simulink model "Modelo_Cinematico_Spline"  (R2020b)
settings: Solver=VariableStepAuto  StartTime=0.0  StopTime=290  RelTol=1e-3
undefined symbols (not defined in the file or in its folder): magnitude
libraries: simulink x2
settings Model: Creator=danie  LastModifiedBy=danie

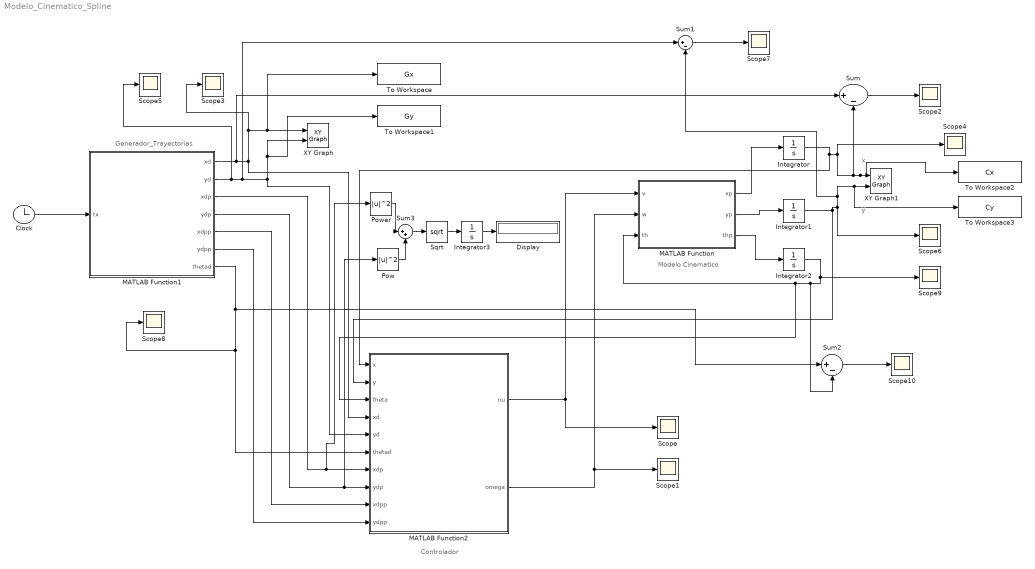
== system Modelo_Cinematico_Spline ==
  note: y
  note: x
  note: Controlador
  note: Generador_Trayectorias
  note: Modelo Cinematico
  Clock : Clock
  Display : Display
  Integrator : Integrator  InitialCondition=50.0557
  Integrator1 : Integrator  InitialCondition=50.0866
  Integrator2 : Integrator
  Integrator3 : Integrator
  MATLAB Function : MATLAB Function  TreatAsAtomicUnit=on
  MATLAB Function1 : MATLAB Function  TreatAsAtomicUnit=on
  MATLAB Function2 : MATLAB Function  TreatAsAtomicUnit=on
  Pow : Math  Operator=magnitude^2  SignedPower=on  RndMeth=Zero  SaturateOnIntegerOverflow=on
  Power : Math  Operator=magnitude^2  SaturateOnIntegerOverflow=on
  Scope{,1..10} (11 alike) : Scope
  Sqrt : Sqrt  SaturateOnIntegerOverflow=on
  Sum : Sum  Inputs=|+-
  Sum1 : Sum  Inputs=|+-
  Sum2 : Sum  Inputs=|+-
  Sum3 : Sum  Inputs=|++
  To Workspace : ToWorkspace  VariableName=Gx  SampleTime=-1
  To Workspace1 : ToWorkspace  VariableName=Gy  SampleTime=-1
  To Workspace2 : ToWorkspace  VariableName=Cx  SampleTime=-1
  To Workspace3 : ToWorkspace  VariableName=Cy  SampleTime=-1
  XY Graph : simulink/Sinks/XY Graph  xmin=0  xmax=100  ymin=0  ymax=100  st=-1
  XY Graph1 : simulink/Sinks/XY Graph  xmin=0  xmax=100  ymin=0  ymax=100  st=-1
  wires:
  MATLAB Function/3(thp) -> Integrator2/1
  Integrator2/1 -> Sum2/2, MATLAB Function2/3(theta), MATLAB Function/3(th), Scope9/1
  MATLAB Function/1(xp) -> Integrator/1
  MATLAB Function/2(yp) -> Integrator1/1
  MATLAB Function2/1(nu) -> MATLAB Function/1(v), Scope/1
  MATLAB Function2/2(omega) -> MATLAB Function/2(w), Scope1/1
  Integrator/1 -> MATLAB Function2/1(x), To Workspace2/1, XY Graph1/1, Sum/2, Scope4/1
  Integrator1/1 -> Scope6/1, Sum1/2, To Workspace3/1, XY Graph1/2, MATLAB Function2/2(y)
  MATLAB Function1/1(xd) -> Sum/1, MATLAB Function2/4(xd), Scope3/1, To Workspace/1, XY Graph/1
  MATLAB Function1/2(yd) -> Scope5/1, Sum1/1, To Workspace1/1, XY Graph/2, MATLAB Function2/5(yd)
  MATLAB Function1/3(xdp) -> Power/1, MATLAB Function2/7(xdp)
  MATLAB Function1/4(ydp) -> Pow/1, MATLAB Function2/8(ydp)
  MATLAB Function1/5(xdpp) -> MATLAB Function2/9(xdpp)
  MATLAB Function1/6(ydpp) -> MATLAB Function2/10(ydpp)
  MATLAB Function1/7(thetad) -> Sum2/1, Scope8/1, MATLAB Function2/6(thetad)
  Clock/1 -> MATLAB Function1/1(tx)
  Sum/1 -> Scope2/1
  Sum1/1 -> Scope7/1
  Sum2/1 -> Scope10/1
  Sum3/1 -> Sqrt/1
  Sqrt/1 -> Integrator3/1
  Integrator3/1 -> Display/1
  Power/1 -> Sum3/1
  Pow/1 -> Sum3/2

== matlab function Modelo_Cinematico_Spline/MATLAB Function1 ==
  data: xd output; yd output; tx input; xdp output; ydp output; xdpp output; ydpp output; thetad output
function [xd, yd, xdp, ydp, xdpp, ydpp, thetad] = fcn(tx)

tmax=300;

xd=(5383481803376765*sin((28386324213466055*((2*pi*tx)/tmax))/9007199254740992))/1125899906842624 - (2564781378595497*cos((28386324213466055*((2*pi*tx)/tmax))/9007199254740992))/18014398509481984 + (4975098477569247*cos((5677264842693211*((2*pi*tx)/tmax))/9007199254740992))/140737488355328 - (5532462661087593*cos((5677264842693211*((2*pi*tx)/tmax))/4503599627370496))/2251799813685248 - (4982669448405143*cos((5677264842693211*((2*pi*tx)/tmax))/2251799813685248))/281474976710656 + (6597269238774799*sin((5677264842693211*((2*pi*tx)/tmax))/9007199254740992))/562949953421312 + (7427178311913285*sin((5677264842693211*((2*pi*tx)/tmax))/4503599627370496))/2251799813685248 + (1488767062451517*sin((5677264842693211*((2*pi*tx)/tmax))/2251799813685248))/281474976710656 - (2110113036993915*cos((17031794528079633*((2*pi*tx)/tmax))/9007199254740992))/140737488355328 - (6032332211127941*sin((17031794528079633*((2*pi*tx)/tmax))/9007199254740992))/281474976710656 + 50;

yd=(2688302397518191*cos((10047744804514215*((2*pi*tx)/tmax))/4503599627370496))/281474976710656 - (773246555679083*sin((10047744804514215*((2*pi*tx)/tmax))/4503599627370496))/35184372088832 + (2417259064448069*cos((16746241340857025*((2*pi*tx)/tmax))/4503599627370496))/281474976710656 + (1557044084674199*sin((16746241340857025*((2*pi*tx)/tmax))/4503599627370496))/1125899906842624 - (826401745574083*cos((3349248268171405*((2*pi*tx)/tmax))/4503599627370496))/140737488355328 - (2589504683792575*cos((3349248268171405*((2*pi*tx)/tmax))/2251799813685248))/140737488355328 + (7002517856441785*cos((3349248268171405*((2*pi*tx)/tmax))/1125899906842624))/1125899906842624 - (5133657206379779*sin((3349248268171405*((2*pi*tx)/tmax))/4503599627370496))/1125899906842624 + (1324039837451005*sin((3349248268171405*((2*pi*tx)/tmax))/2251799813685248))/281474976710656 + (6400066323978353*sin((3349248268171405*((2*pi*tx)/tmax))/1125899906842624))/562949953421312 + 50;

xdp=(37454444707077569124597075189589*pi*cos((5677264842693211*pi*tx)/(4503599627370496*tmax)))/(2535301200456458802993406410752*tmax) + (42166058310638804388005690208135*pi*cos((5677264842693211*pi*tx)/(2251799813685248*tmax)))/(5070602400912917605986812821504*tmax) + (8452124902615645497794392551087*pi*cos((5677264842693211*pi*tx)/(1125899906842624*tmax)))/(316912650057057350374175801344*tmax) - (6421340171565460806896461762357*pi*cos((1064487158004977*pi*tx)/(281474976710656*tmax)))/(79228162514264337593543950336*tmax) - (28244951675640404604248229282117*pi*sin((5677264842693211*pi*tx)/(4503599627370496*tmax)))/(633825300114114700748351602688*tmax) + (31409255759305517195060497431123*pi*sin((5677264842693211*pi*tx)/(2251799813685248*tmax)))/(5070602400912917605986812821504*tmax) + (28287934082192092596880783584173*pi*sin((5677264842693211*pi*tx)/(1125899906842624*tmax)))/(316912650057057350374175801344*tmax) + (2246188229818903474228688714955*pi*sin((1064487158004977*pi*tx)/(281474976710656*tmax)))/(39614081257132168796771975168*tmax) + (19102157483493471684558188323605*pi*cos((3548290526683257*pi*tx)/(562949953421312*tmax)))/(633825300114114700748351602688*tmax) + (9100589468684026021756445493729*pi*sin((3548290526683257*pi*tx)/(562949953421312*tmax)))/(10141204801825835211973625643008*tmax);

ydp=(407416187817311810543913761309*pi*cos((261660020950891*pi*tx)/(35184372088832*tmax)))/(39614081257132168796771975168*tmax) - (632500057447212912553468779479*pi*sin((261660020950891*pi*tx)/(35184372088832*tmax)))/(9903520314283042199192993792*tmax) - (17193892507853127879432298019495*pi*cos((3349248268171405*pi*tx)/(2251799813685248*tmax)))/(2535301200456458802993406410752*tmax) + (4434538132572727079447629512025*pi*cos((3349248268171405*pi*tx)/(1125899906842624*tmax)))/(316912650057057350374175801344*tmax) + (21435411051766629023004113595965*pi*cos((3349248268171405*pi*tx)/(562949953421312*tmax)))/(316912650057057350374175801344*tmax) + (2767824615177823544638369696615*pi*sin((3349248268171405*pi*tx)/(2251799813685248*tmax)))/(316912650057057350374175801344*tmax) + (8672894077614023540335566317875*pi*sin((3349248268171405*pi*tx)/(1125899906842624*tmax)))/(158456325028528675187087900672*tmax) - (23453170803526987627261784157925*pi*sin((3349248268171405*pi*tx)/(562949953421312*tmax)))/(633825300114114700748351602688*tmax) - (971173007804127331951225917991*pi*cos((1255968100564277*pi*tx)/(281474976710656*tmax)))/(9903520314283042199192993792*tmax) - (3376422055953314277671472262907*pi*sin((1255968100564277*pi*tx)/(281474976710656*tmax)))/(79228162514264337593543950336*tmax);

xdpp=(32291535398964944679140506992381246790162795353*pi^2*cos((3548290526683257*pi*tx)/(562949953421312*tmax)))/(5708990770823839524233143877797980545530986496*tmax^2) - (67780004437891569776866379107147617745651381485*pi^2*sin((3548290526683257*pi*tx)/(562949953421312*tmax)))/(356811923176489970264571492362373784095686656*tmax^2) - (160354071131681968090375756460233262699399607687*pi^2*cos((5677264842693211*pi*tx)/(4503599627370496*tmax)))/(2854495385411919762116571938898990272765493248*tmax^2) + (178318663457464468702307355009051006962292205953*pi^2*cos((5677264842693211*pi*tx)/(2251799813685248*tmax)))/(11417981541647679048466287755595961091061972992*tmax^2) + (160598093637252212663730214209012445414834149503*pi^2*cos((5677264842693211*pi*tx)/(1125899906842624*tmax)))/(356811923176489970264571492362373784095686656*tmax^2) + (2391038525104154692777831774840356231624331035*pi^2*cos((1064487158004977*pi*tx)/(281474976710656*tmax)))/(11150372599265311570767859136324180752990208*tmax^2) - (212638802138088304827737641160315177219188180279*pi^2*sin((5677264842693211*pi*tx)/(4503599627370496*tmax)))/(11417981541647679048466287755595961091061972992*tmax^2) - (239387880401941574160516267743202310404541471485*pi^2*sin((5677264842693211*pi*tx)/(2251799813685248*tmax)))/(11417981541647679048466287755595961091061972992*tmax^2) - (47984951555671583979630787606204462637985570357*pi^2*sin((5677264842693211*pi*tx)/(1125899906842624*tmax)))/(356811923176489970264571492362373784095686656*tmax^2) + (6835434149812908795327482680102998001597250789*pi^2*sin((1064487158004977*pi*tx)/(281474976710656*tmax)))/(22300745198530623141535718272648361505980416*tmax^2);

ydpp=(1219762317931045568593540067381353994426207507*pi^2*sin((1255968100564277*pi*tx)/(281474976710656*tmax)))/(2787593149816327892691964784081045188247552*tmax^2) - (4240678396319015130497079762907630620796373239*pi^2*cos((1255968100564277*pi*tx)/(281474976710656*tmax)))/(22300745198530623141535718272648361505980416*tmax^2) - (165499978283077491769036625538731210767565789*pi^2*cos((261660020950891*pi*tx)/(35184372088832*tmax)))/(348449143727040986586495598010130648530944*tmax^2) - (106604528240009950942948130502300866584876319*pi^2*sin((261660020950891*pi*tx)/(35184372088832*tmax)))/(1393796574908163946345982392040522594123776*tmax^2) + (9270131798986510997054235237400213970668294075*pi^2*cos((3349248268171405*pi*tx)/(2251799813685248*tmax)))/(713623846352979940529142984724747568191373312*tmax^2) + (29047675469482803324353555333873198935215364375*pi^2*cos((3349248268171405*pi*tx)/(1125899906842624*tmax)))/(178405961588244985132285746181186892047843328*tmax^2) - (78550491696840922343442503487770950837489134625*pi^2*cos((3349248268171405*pi*tx)/(562949953421312*tmax)))/(356811923176489970264571492362373784095686656*tmax^2) + (57586614705052384093879702349227552026691540475*pi^2*sin((3349248268171405*pi*tx)/(2251799813685248*tmax)))/(5708990770823839524233143877797980545530986496*tmax^2) - (14852369160659262563490299824908137359208645125*pi^2*sin((3349248268171405*pi*tx)/(1125899906842624*tmax)))/(356811923176489970264571492362373784095686656*tmax^2) - (71792513342671577226823118665849048129536380825*pi^2*sin((3349248268171405*pi*tx)/(562949953421312*tmax)))/(178405961588244985132285746181186892047843328*tmax^2);

thetad=atan2(ydp, xdp)+pi; %orientacion nominal

== matlab function Modelo_Cinematico_Spline/MATLAB Function ==
  data: v input; xp output; w input; yp output; thp output; th input
function [xp, yp, thp] = fcn(v, w, th)

xp=v.*cos(th);
yp=v.*sin(th);
thp=w;

== matlab function Modelo_Cinematico_Spline/MATLAB Function2 ==
  data: x input; nu output; omega output; y input; theta input; xd input; yd input; thetad input; xdp input; ydp input; xdpp input; ydpp input
function [nu, omega] = fcn(x, y, theta, xd, yd, thetad, xdp, ydp, xdpp, ydpp)

b=0.0; %grado de libertad adicional
zeta=12; %coeficiente de amortiguamiento

nud=-sqrt(xdp^2+ydp^2); %velocidad lineal deseada
omegad=((ydpp*xdp)-(xdpp*ydp))/(xdp^2+ydp^2); %velocidad angular deseada

k3=2*zeta*sqrt(omegad^2+b*nud^2);
k1=k3;
k2=b*abs(nud);

nu=nud*cos(thetad-theta)+k1*(cos(theta)*(xd-x)+sin(theta)*(yd-y)); %velocidad lineal

omega=omegad+k2*sign(nud)*(cos(theta)*(xd-x)-sin(theta)*(yd-y))+k3*(thetad-theta); %velocidad angular
